simulink library "visionsources"  (R2015b)
settings: Solver=ode45  SolverMode=SingleTasking  StartTime=0.0  StopTime=10.0  RelTol=1e-3
undefined symbols (not defined in the file): checker_board
libraries: dspvision x1
settings Model: ExtModeAutoUpdateStatusClock=off  Creator=The MathWorks, Inc.  LastModifiedBy=The MathWorks, Inc.
settings DataIOCC: SaveFormat=Array  SignalLoggingSaveFormat=ModelDataLogs
settings OptimizationCC: BlockReduction=off  BooleanDataType=off  ExpressionDepthLimit=2147483647
settings DebuggingCC: SaveWithParameterizedLinksMsg=none  UnderspecifiedInitializationDetection=Classic  MergeDetectMultiDrivingBlocksExec=none  SignalResolutionControl=TryResolveAllWithWarning  FcnCallInpInsideContextMsg=UseLocalSettings  StateNameClashWarn=warning  StrictBusMsg=Warning
settings HardwareCC: ProdBitPerPointer=32  ProdLargestAtomicFloat=None  ProdIntDivRoundTo=Undefined  ProdEndianess=Unspecified  ProdWordSize=32  ProdHWDeviceType=32-bit Generic  TargetUnknown=on
settings GRTTargetCC: GeneratePreprocessorConditionals=Disable all  CombineOutputUpdateFcns=off  GRTInterface=on
settings ConfigComp: CovModelRefEnable=Off

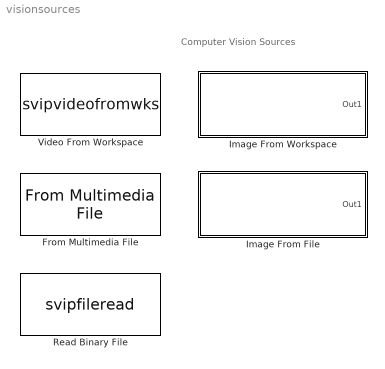
== system visionsources ==
  note: Computer Vision Sources
  From Multimedia File : dspvision/From Multimedia File  inputFilename=vipmen.avi  loop=on  numPlays=inf  outputStreams=Video only  videoDataType=single  audioDataType=int16  inheritSampleTime=on  userDefinedSampleTime=1/30  noAudioOutput=off  isIntensityVideo=off  fourcc=RGB  colorVideoFormat=One multidimensional signal  outputEOF=off  dataOrg=Column-major  audioFrameSize=1024  computeAudioFrameSize=off  outSamplingMode=Sample based
  Image From File : Subsystem  Tag=vipblks_nd  DialogController=vipDDGCreate  mask(Image From File){FileName=peppers.png, imagePorts=One multidimensional signal, Ts=inf, ImageDataType=Inherit from input image, Signed=on, WordLength=16, sdImageDataType=uint(8), FractionLengthMode=User-defined, FractionLength=15, OutPortLabels=R|G|B}
      mask prompts: FileName "File Name:"; imagePorts "Image signal:"; Ts "Sample time:"; ImageDataType "Output data type:"; WordLength "Word length:"; sdImageDataType "User-defined data type (e.g. sfix(16), uint(8), float('single')):"; FractionLengthMode "Set fraction length in output to:"; FractionLength "Fraction length:"; OutPortLabels "Output port labels:"
      mask help:
      | Reads an image from a file.
      |
      | Use the File name parameter to specify the image file you want to import into your model. Use the Sample time parameter to set the sample period of the block.
      mask init:
      | vipblks_nd_compatible;
      | [v, namechange]=vipblkimsrc(1, '',0,FileName);
      | ImageValue = v;
      | vipblkimsrc(2, v, namechange,FileName);
      mask Help: eval('visionblockhelp;')
      mask TypeOptions imagePorts: One multidimensional signal | Separate color signals
      mask Callback imagePorts: vipblkimsrc(-1);
      mask TypeOptions ImageDataType: double | single | int8 | uint8 | int16 | uint16 | int32 | uint32 | boolean | Fixed-point | User-defined | Inherit from input image | Inherit via back propagation
      mask TypeOptions FractionLengthMode: Best precision | User-defined
      mask Display: disp('peppers.png');port_label('output',1,'Image');
  Image From Workspace : Subsystem  Tag=vipblks_nd  mask(Image From Workspace){ImageValue=checker_board(10), Ts=inf, imagePorts=One multidimensional signal, ImageDataType=Inherit from 'Value', Signed=on, WordLength=16, sdImageDataType=sfix(16), FractionLengthMode=User-defined, FractionLength=15, OutPortLabels=R|G|B}
      mask prompts: ImageValue "Value:"; Ts "Sample time:"; imagePorts "Image signal:"; ImageDataType "Output data type:"; WordLength "Word length:"; sdImageDataType "User-defined data type (e.g. sfix(16), uint(8), float('single')):"; FractionLengthMode "Set fraction length in output to:"; FractionLength "Fraction length:"; OutPortLabels "Output port labels:"
      mask help:
      | Imports an image from the MATLAB workspace.
      |
      | Use the Value parameter to specify the MATLAB workspace variable that contains or an expression that specifies the image you want to import into your model. Use the Sample time parameter to set the sample period of the block.
      mask init:
      | ImageVal = get_param(gcbh, 'ImageValue');
      | vipblks_nd_compatible;
      | [v,namechange]=vipblkimsrc(1, ImageValue, 0,'');
      | vipblkimsrc(2, v, namechange,'');
      mask Help: eval('visionblockhelp;')
      mask TypeOptions imagePorts: One multidimensional signal | Separate color signals
      mask Callback imagePorts: vipblkimsrc(-1);
      mask TypeOptions ImageDataType: double | single | int8 | uint8 | int16 | uint16 | int32 | uint32 | boolean | Fixed-point | User-defined | Inherit from 'Value' | Inherit via back propagation
      mask Callback ImageDataType: vipblkimsrc(-1, 1);
      mask Callback sdImageDataType: vipblkimsrc(-1);
      mask TypeOptions FractionLengthMode: Best precision | User-defined
      mask Callback FractionLengthMode: vipblkimsrc(-1, 1);
      mask Display: disp(ImageVal);port_label('output',1,'Image');
  Read Binary File : S-Function  DialogController=vipDDGCreate  FunctionName=svipfileread  Parameters=FileName, loopOrNot, numLoops, VideoFormat, FOURCC, BitStreamFormat, NumOutputs, Bits, ComponentOrder, Interlaced, LineOrdering, FrameSizes, PackFrameSize, SignedOutput, FileEndian, OutputEOF,Ts  SFunctionDeploymentMode=off  EnableBusSupport=off  mask(Read Binary File){FileName=vipmen.bin, loopOrNot=on, numLoops=1, VideoFormat=Four character codes, FOURCC=I420, BitStreamFormat=Planar, NumOutputs=3, ComponentOrder=[1 2 3], Interlaced=off, LineOrdering=Top line first, Ts=1/30, Component1=Y', Component2=Cb, Component3=Cr, Component4=Alpha, Bits1=8, Bits2=8, Bits3=8, Bits4=8, Rows1=120, Rows2=60, Rows3=60, Rows4=288, Cols1=160, Cols2=80, Cols3=80, Cols4=352, YRows=120, YCols=160, SignedOutput=off, FileEndian=Little endian, OutputEOF=off}
      mask prompts: FileName "File name:"; loopOrNot "Loop"; numLoops "Number of times to play file:"; VideoFormat "Video format:"; FOURCC "Video file format label:"; BitStreamFormat "Bit stream format:"; NumOutputs "Number of outputs:"; ComponentOrder "Component order in bit stream, e.g. Y' | Cb | Cr:"; Interlaced "Interlaced video"; LineOrdering "Line ordering:"; Ts "Sample time:"; YRows "Size of Y' compoenet Rows:"; YCols "Size of Y' component Cols:"; SignedOutput "Input file has signed data:"; FileEndian "Byte order in binary file:"; OutputEOF "Output end-of-file indicator:"
      mask help: Read binary video data from file in the specified format.
      mask init:
      | Rows = {Rows1 Rows2 Rows3 Rows4};
      | Cols = {Cols1 Cols2 Cols3 Cols4};
      | Bits = {Bits1 Bits2 Bits3 Bits4};
      | Components = {Component1 Component2 Component3 Component4};
      | videoformat = get_param(gcb, 'VideoFormat');
      | bitstreamformat = get_param(gcb, 'BitStreamFormat');
      | fourcc = get_param(gcb, 'FOURCC');
      | outputeof = get_param(gcb, 'OutputEOF');
      | [FrameSizes, PackFrameSize, FOURCC, NumOutputs,...
      |     maskdisplay, Bits, FileName] =...
      |     vipblkreadbinaryfile(NumOutputs, Components, ComponentOrder,...
      |     Rows, Cols, YRows, YCols, Bits, FileName, videoformat, ...
      |     bitstreamformat, fourcc, outputeof);
      | ComponentOrder = ComponentOrder - 1;
      | set_param(gcb, 'MaskDisplay', maskdisplay);
      mask Help: eval('visionblockhelp;')
      mask TypeOptions VideoFormat: Four character codes | Custom
      mask TypeOptions FOURCC: AYUV | CLJR | cyuv | GREY | I420 | IF09 | IMC1 | IMC2 | IMC3 | IMC4 | IUYV | IY41 | IYU1 | IYU2 | IYUV | NV12 | NV21 | UYNV | UYVY | V210 | Y411 | Y41P | Y41T | Y422 | Y42T | Y8 | Y800 | YUNV | YUY2 | YUYV | YV12 | YV16 | YVU9 | YVYU
      mask TypeOptions BitStreamFormat: Packed | Planar
      mask TypeOptions NumOutputs: 1 | 2 | 3 | 4
      mask TypeOptions LineOrdering: Top line first | Bottom line first
      mask TypeOptions FileEndian: Little endian | Big endian
      mask Display: disp('vipmen.bin');port_label('output', 1,'Y''');port_label('output', 2,'Cb');port_label('output', 3,'Cr');
  Video From Workspace : S-Function  FunctionName=svipvideofromwks  Parameters=signal,Ts, finaloutActive,imagePorts, finalout  SFunctionDeploymentMode=off  EnableBusSupport=off  mask(Video From Workspace){signal=rand(32,32,3,5), Ts=1, finalout=Obsolete, finaloutActive=Cyclic repetition, imagePorts=One multidimensional signal, OutPortLabels=R|G|B}
      mask prompts: Ts "Sample time:"; finalout "Form output after final value by (obsoleted):"; finaloutActive "Form output after final value by:"; imagePorts "Image signal:"; OutPortLabels "Output port labels:"
      mask help:
      | Outputs video frames from the MATLAB workspace at successive sample times.
      |
      | If the video signal is a M-by-N-by-T workspace array, the block outputs an intensity video signal, where M and N are the number of rows and columns in a single video frame, and T is the number of frames in the video signal.
      |
      | If the video signal is a M-by-N-by-C-by-T workspace array, the block outputs a color video signal, where M and N are the number of rows and columns in a single video frame, C is the number of outputs from the block, and T is the number of frames in the video stream.
      mask init:
      | signalValue = get_param(gcbh, 'signal');
      | vipblkvideofromws(signal);
      mask Help: eval('visionblockhelp;')
      mask TypeOptions finalout: Setting to zero | Holding final value | Cyclic repetition | Obsolete
      mask TypeOptions finaloutActive: Setting to zero | Holding final value | Cyclic repetition
      mask TypeOptions imagePorts: One multidimensional signal | Separate color signals
      mask Callback imagePorts: vipblkvideofromws
      mask Display:
      | disp(get_param(gcbh, 'signal'));
      | port_label('output',1,'Image');

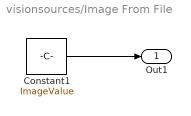
== system visionsources/Image From File ==
  Constant1 : Constant  Value=ImageValue  SampleTime=Ts
  Out1 : Outport
  wires:
  Constant1/1 -> Out1/1

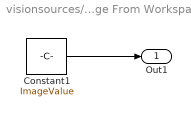
== system visionsources/Image From Workspace ==
  Constant1 : Constant  Value=ImageValue  SampleTime=Ts
  Out1 : Outport
  wires:
  Constant1/1 -> Out1/1
